simulink model "c230403_FCEV_SLMP_SQP"  (R2022b)
settings: Solver=FixedStepAuto  StartTime=0.0  StopTime=DrvCycLen  FixedStep=1  RelTol=1e-3
values from neighbouring files (symbols this model uses):
  AccThrshd = 1    [Config_c221112.m]    (also in Config_c221127.m; Config_c221218.m; Config_c230117.m; Config_c230321.m)
  AlphaRampFactor = 8    [Config_c221112.m]    (also in Config_c221127.m; Config_c221218.m; Config_c230117.m; Config_c230321.m)
  Bat_ori_SOC2 = [0 0.001 0.002 0.003 0.004 0.005 0.006 0.007 0.008 0.009 0.01 0.011 ... (1001 elements, 1x1001)]    [FCEV_original_data.mat]
  Bat_ori_Uoc_chg_V = [2.4478 2.54923264342 2.6007 2.6383 2.66953057366 2.69636321708 2.7197 2.74042850391 2.75906114733 2.77619379074 2.792 2.80675907757 ... (1001 elements, 1x1001)]    [FCEV_original_data.mat]
  Bat_ori_Uoc_dis_V = [1.9998 2.03916768329 2.24724374236 2.39700902919 2.48767431602 2.5476 2.5882 2.6202 2.64771773167 2.6719 2.6933 2.71251566192 ... (1001 elements, 1x1001)]    [FCEV_original_data.mat]
  Bat_power_max_kW = 50    [FCEV_original_data.mat]
  Bat_power_min_kW = 0    [FCEV_original_data.mat]
  Bat_SOC_min = 0.3    [FCEV_original_data.mat]
  BattOnly = 0    [Config_c221218.m]    (also in Config_c230117.m = BattSocRightNow > BattSocLowerLimit; Config_c230321.m = double(BattSocRightNow > BattSocLowerLimit))
  BattPack_current = BattCell_current * 9    (= 20.7)    [Config_c230321.m]
  BattSocInit = 0.9    [Config_c221112.m]    (also in Config_c221127.m = 0.3; Config_c221218.m = 0.3; Config_c230117.m = 0.8; Config_c230321.m = 0.8)
  BattSocLowerLimit = 0.25    [Config_c221112.m]    (also in Config_c221127.m = 0.3; Config_c221218.m = 0.3; Config_c230117.m = 0.3; Config_c230321.m = 0.3)
  BattSocRightNow = BattSocRightNow - SocDrop    [Config_c221218.m]    (also in Config_c230117.m; Config_c230321.m)
  BattSocUpperLimit = 0.9    [Config_c221112.m]    (also in Config_c221127.m = 0.8; Config_c221218.m = 0.8; Config_c230117.m = 0.8; Config_c230321.m = 0.8)
  CFWF = 0.5    [Config_c221127.m]    (also in Config_c221218.m; Config_c230117.m; Config_c230321.m)
  DCAC_eff = 0.95    [FCEV_original_data.mat]
  DCDC_ori_eff = [0.95 0.96 0.97 0.976 0.98 0.978 0.973 0.962]    [FCEV_original_data.mat]
  DCDC_ori_power_kW = [0 10 20 30 40 50 60 70]    [FCEV_original_data.mat]
  DeAccThrshd = -1    [Config_c221112.m]    (also in Config_c221127.m; Config_c221218.m; Config_c230117.m; Config_c230321.m)
  DeltaFcPwrRcm_down = 0.5    [Config_c221127.m]    (also in Config_c221218.m; Config_c230117.m; Config_c230321.m)
  DeltaFcPwrRcm_up = 2    [Config_c221127.m]    (also in Config_c221218.m = 3; Config_c230117.m = 4; Config_c230321.m = 4)
  DrvCycRange = sum(DrvCycVps(:,2))    [Config_c221112.m]    (also in Config_c221127.m; Config_c221218.m; Config_c230117.m; Config_c230321.m)
  FC_ori_eff = [0.1 0.33 0.492 0.533 0.559 0.596 0.591 0.562 0.508]    [FCEV_original_data.mat]
  FC_ori_fuel_rate_gps = [0 0.0505050505051 0.0846883468835 0.117260787992 0.149075730471 0.279642058166 0.423011844332 0.593119810202 0.820209973753]    [FCEV_original_data.mat]
  FC_ori_power_kW = [0 2 5 7.5 10 20 30 40 50]    [FCEV_original_data.mat]
  FC_power_max_kW = 50    [FCEV_original_data.mat]
  FC_power_min_kW = 0    [FCEV_original_data.mat]
  FcPwrDropCall = 6    [Config_c221127.m]    (also in Config_c221218.m; Config_c230117.m; Config_c230321.m)
  HydpriceRmb = 30    [Config_c221127.m]    (also in Config_c221218.m; Config_c230117.m; Config_c230321.m)
  m = Time_sample    [Config_c22100601.m]    (also in Config_c22100701.m)
  MC_eff_brk_average = 0.810578512397    [FCEV_original_data.mat]
  MC_eff_dri_average = 0.810578512397    [FCEV_original_data.mat]
  MC_inertia = 0.06    [FCEV_original_data.mat]
  MC_ori_eff = [0.7 0.78 0.85 0.86 0.81 0.82 0.79 0.78 0.78 0.78 0.78 0.7 ... (231 elements, 11x21)]    [FCEV_original_data.mat]
  MC_ori_power_brk_req_kW = [0 -28.3912930389 -56.7825860779 -85.1738791168 -113.565172156 -141.956465195 -170.347758234 -198.739051273 -227.130344311 -255.52163735 -283.912930389 0 ... (121 elements, 11x11)]    [FCEV_original_data.mat]
  MC_ori_power_dri_req_kW = [0 0 0 0 0 0 0 0 0 0 0 0 ... (121 elements, 11x11)]    [FCEV_original_data.mat]
  MC_ori_spd_rpm = [0 1000 2000 3000 4000 5000 6000 7000 8000 9000 10000]    [FCEV_original_data.mat]
  MC_ori_trq_brk_max_Nm = [-271.1368 -271.1368 -271.1368 -237.5159 -178.1369 -142.4824 -118.7579 -101.8119 -89.0685 -79.172 -71.1734]    [FCEV_original_data.mat]
  MC_ori_trq_brk_Nm = [-271.136848522 -244.02316367 -216.909478817 -189.795793965 -162.682109113 -135.568424261 -108.454739409 -81.3410545565 -54.2273697044 -27.1136848522 0]    [FCEV_original_data.mat]
  MC_ori_trq_dri_max_Nm = [271.1368 271.1368 271.1368 237.5159 178.1369 142.4824 118.7579 101.8119 89.0685 79.172 71.1734]    [FCEV_original_data.mat]
  MC_ori_trq_dri_Nm = [0 27.1136848522 54.2273697044 81.3410545565 108.454739409 135.568424261 162.682109113 189.795793965 216.909478817 244.02316367 271.136848522]    [FCEV_original_data.mat]
  MC_ori_trq_Nm = [-271.136848522 -244.02316367 -216.909478817 -189.795793965 -162.682109113 -135.568424261 -108.454739409 -81.3410545565 -54.2273697044 -27.1136848522 0 27.1136848522 ... (21 elements, 1x21)]    [FCEV_original_data.mat]
  MC_power_max_kW = 75    [FCEV_original_data.mat]
  MC_spd_max_rpm = 10000    [FCEV_original_data.mat]
  MC_spd_min_rpm = 0    [FCEV_original_data.mat]
  MC_spd_scale = 1    [FCEV_original_data.mat]
  MC_trq_scale = 1    [FCEV_original_data.mat]
  nbl_std = (20/nbl_btm)^(1/0.57)    [Config_c230321.m]
  no_FcPwrSlowDrop = 1    [Config_c230321.m]
  Placeholder = 0    [Config_c221127.m]    (also in Config_c221218.m; Config_c230117.m; Config_c230321.m)
  PredLen = 5    [Config_c221112.m]    (also in Config_c221127.m; Config_c221218.m; Config_c230117.m; Config_c230321.m)
  Q_batt = 20.7*3600    (= 74520)    [Config_c22100701.m]    (also in Config_c230321.m = 18000)
  Road_u = 0.75    [FCEV_original_data.mat]
  SC_np = 1    [Config_c230321.m]
  SC_ns = 100    [Config_c230321.m]
  SC_rc = 1000    [Config_c230321.m]
  SLMP_LearningRate = 0.05    [Config_c221112.m]    (also in Config_c221127.m; Config_c221218.m; Config_c230117.m; Config_c230321.m)
  tDegTable = [zeros(1,3),linspace(0,0.13,47)]    [Config_c221127.m]    (also in Config_c221218.m; Config_c230117.m; Config_c230321.m)
  usd2rmb = 7.116    [Config_c22100601.m]    (also in Config_c22100701.m; Config_c221106.m = 6; Config_c221112.m = 6; Config_c221127.m = 6)
  Veh_air_density_kgpm2 = 1.2    [FCEV_original_data.mat]
  Veh_brk_front = [1 0.6 0.608 0.61 0.618 0.624 0.636 0.645 0.655]    [FCEV_original_data.mat]
  Veh_brk_z = [0.1 0.2 0.3 0.4 0.5 0.6 0.7 0.8 0.9]    [FCEV_original_data.mat]
  Veh_brk_z_max = 0.7    [FCEV_original_data.mat]
  Veh_brk_z_min = 0.1    [FCEV_original_data.mat]
  Veh_coeff_drag = 0.312    [FCEV_original_data.mat]
  Veh_coeff_roll = 0.00863    [FCEV_original_data.mat]
  Veh_final_drive_inertia = 0.1105    [FCEV_original_data.mat]
  Veh_final_drive_ratio = 3.47    [FCEV_original_data.mat]
  Veh_frontal_area_m2 = 2.06    [FCEV_original_data.mat]
  Veh_gravity_acc_ms2 = 9.81    [FCEV_original_data.mat]
  Veh_mass_cargo_kg = 113    [FCEV_original_data.mat]
  Veh_mass_curb_kg = 1157    [FCEV_original_data.mat]
  Veh_mech_eff = 0.9    [FCEV_original_data.mat]
  Veh_rotary_mass_conversion_factor = 1.05    [FCEV_original_data.mat]
  Veh_size_cg_height_m = 0.53    [FCEV_original_data.mat]
  Veh_wheel_inertia = 3.1039    [FCEV_original_data.mat]
  Veh_wheel_radius_m = 0.313    [FCEV_original_data.mat]
  Veh_wt_frac_front = 0.5    [FCEV_original_data.mat]
  VstdThrshd = 2    [Config_c221112.m]    (also in Config_c221127.m; Config_c221218.m; Config_c230117.m; Config_c230321.m)
undefined symbols (not defined in the file or in its folder): Bat_ori_temp, SC_iv, SC_nm, SC_SocTable
libraries: autolibshared x2
(part 7 of 7)

== system c230403_FCEV_SLMP_SQP/Subsystem4/VehModel_Pred+9/车轮模型/Interia torque1 ==
  note: This block computes the torque required to overcome the inertia of the
      | wheels and axle.
  车轮线速度 m/s : Inport
  Add : Sum  Inputs=+-
  Add1 : Sum  Inputs=+-
  Clock : Clock
  Constant : Constant  Value=Veh_wheel_inertia
  Constant2 : Constant  Value=0
  Divide : Product  Inputs=**/
  Memory : Memory  InheritSampleTime=on
  Memory1 : Memory  InheritSampleTime=on
  Saturation : Saturate  UpperLimit=1.1  LowerLimit=0.9
  Switch : Switch  SaturateOnIntegerOverflow=off  InputSameDT=off
  axle input speed (rad/s) : Gain  Gain=1/Veh_wheel_radius_m
  inertia torque (Nm) : Outport  InitialOutput=0
  wires:
  Divide/1 -> inertia torque (Nm)/1
  车轮线速度 m/s/1 -> axle input speed (rad/s)/1
  Saturation/1 -> Divide/3
  Add1/1 -> Saturation/1
  Constant2/1 -> Switch/1
  axle input speed (rad/s)/1 -> Add/1, Memory/1
  Memory/1 -> Add/2
  Clock/1 -> Add1/1, Memory1/1
  Memory1/1 -> Add1/2
  Constant/1 -> Divide/2
  Add/1 -> Switch/3, Switch/2
  Switch/1 -> Divide/1

== system c230403_FCEV_SLMP_SQP/Subsystem4/VehModel_Pred+9/驱动电机模型/Brake torque_limited ==
  tor_req nm : Inport
  mc spd rpm : Inport  Port=2
  1-D Lookup Table : Lookup_n-D  NumberOfTableDimensions=1  BreakpointsForDimension1=MC_ori_spd_rpm  Table=MC_ori_trq_brk_max_Nm  RndMeth=Simplest
  MinMax : MinMax  Function=max  Inputs=2
  limted mc torque nm : Outport
  wires:
  MinMax/1 -> limted mc torque nm/1
  1-D Lookup Table/1 -> MinMax/2
  mc spd rpm/1 -> 1-D Lookup Table/1
  tor_req nm/1 -> MinMax/1

== system c230403_FCEV_SLMP_SQP/Subsystem4/VehModel_Pred+9/驱动电机模型/Drive torque_limited ==
  tor_req nm : Inport
  mc spd rpm : Inport  Port=2
  1-D Lookup Table : Lookup_n-D  NumberOfTableDimensions=1  BreakpointsForDimension1=MC_ori_spd_rpm  Table=MC_ori_trq_dri_max_Nm  RndMeth=Simplest
  MinMax : MinMax  Inputs=2
  limted mc torque nm : Outport
  wires:
  MinMax/1 -> limted mc torque nm/1
  1-D Lookup Table/1 -> MinMax/2
  mc spd rpm/1 -> 1-D Lookup Table/1
  tor_req nm/1 -> MinMax/1

== system c230403_FCEV_SLMP_SQP/Subsystem4/VehModel_Pred+9/驱动电机模型/Inertia torque ==
  motor spd rpm : Inport
  Derivative : Derivative
  Gain1 : Gain  Gain=MC_inertia
  rpm->rad/s : Gain  Gain=2*pi/60
  Out1 : Outport
  wires:
  motor spd rpm/1 -> rpm->rad/s/1
  rpm->rad/s/1 -> Derivative/1
  Gain1/1 -> Out1/1
  Derivative/1 -> Gain1/1

== system c230403_FCEV_SLMP_SQP/Subsystem4/VehModel_Pred+9/驱动电机模型/Inertia torque1 ==
  motor spd rpm : Inport
  Derivative : Derivative
  Gain1 : Gain  Gain=MC_inertia
  rpm->rad/s : Gain  Gain=2*pi/60
  Out1 : Outport
  wires:
  motor spd rpm/1 -> rpm->rad/s/1
  rpm->rad/s/1 -> Derivative/1
  Gain1/1 -> Out1/1
  Derivative/1 -> Gain1/1

== system c230403_FCEV_SLMP_SQP/VehModel_Current/车轮模型/Regenerative energy compute/compute of the brk energy ==
  motor brk force in front wheel N : Inport
  wheel linear spd m/s : Inport  Port=2
  Add : Sum
  Gain1 : Gain  Gain=-1
  Memory1 : Memory  InheritSampleTime=on
  Product : Product  RndMeth=Zero
  Scope : Scope
  Ws->kWh : Gain  Gain=1/(1000*3600)
  制动能量 : ToWorkspace  VariableName=Energy_regenerative_brk_kWh  SaveFormat=Timeseries  SampleTime=-1
  "regenerative brk energy kwh " : Outport
  wires:
  motor brk force in front wheel N/1 -> Product/1
  wheel linear spd m/s/1 -> Product/2
  Product/1 -> Gain1/1
  Ws->kWh/1 -> Scope/1, 制动能量/1, "regenerative brk energy kwh "/1
  Add/1 -> Memory1/1, Ws->kWh/1
  Memory1/1 -> Add/2
  Gain1/1 -> Add/1

== matlab function c230403_FCEV_SLMP_SQP/SuperCapacitor/MATLAB Function1 ==
  data: P input; y output; n input; c input; u_k input
function y = fcn(P,n,c,u_k)

y = (2*P/(n*c)+(u_k)^2)^(1/2);

== matlab function c230403_FCEV_SLMP_SQP/MATLAB Function ==
  data: PredLen input; Enable output
function Enable = fcn(PredLen)

u = zeros(9,1);
u(1:PredLen,1) = 1;

Enable = u;

== stateflow chart c230403_FCEV_SLMP_SQP/Chart ==
  state LowSpeed_URBAN
    note: [2,10]
    state LowConditioning
      entry:
      DrvState = 10;
    state LowDeAcc
      entry:
      DrvState = 9;
    state LowAcc
      entry:
      DrvState = 11;
    (default) -> LowConditioning
    LowConditioning -> (junction 81) [order 1] : [a_ave < DeAccThrshd]
    (junction 81) -> LowDeAcc : [v_std > VstdThrshd]
    LowDeAcc -> LowConditioning [order 1] : [a_ave > DeAccThrshd]
    LowDeAcc -> LowConditioning [order 2] : [v_std < VstdThrshd]
    LowConditioning -> (junction 78) [order 2] : [a_ave > AccThrshd]
    (junction 78) -> LowAcc : [v_std > VstdThrshd]
    LowAcc -> LowConditioning [order 2] : [a_ave < AccThrshd]
    LowAcc -> LowConditioning [order 1] : [v_std < VstdThrshd]
  state Init
    entry:
    DrvState = 0;
  state MidSpeed_SUBURB
    note: (10,25]
    state MidDeAcc
      entry:
      DrvState = 19;
    state MidConditioning
      entry:
      DrvState = 20;
    state MidAcc
      entry:
      DrvState = 21;
    (default) -> MidConditioning
    MidConditioning -> (junction 94) [order 1] : [a_ave < DeAccThrshd]
    (junction 94) -> MidDeAcc : [v_std > VstdThrshd]
    MidDeAcc -> MidConditioning [order 2] : [a_ave > DeAccThrshd]
    MidDeAcc -> MidConditioning [order 1] : [v_std < VstdThrshd]
    MidConditioning -> (junction 92) [order 2] : [a_ave > AccThrshd]
    (junction 92) -> MidAcc : [v_std > VstdThrshd]
    MidAcc -> MidConditioning [order 1] : [a_ave < AccThrshd]
    MidAcc -> MidConditioning [order 2] : [v_std < VstdThrshd]
  state HighSpeed_HIGHWAY
    note: (25,inf)
    state HighDeAcc
      entry:
      DrvState = 29;
    state HighConditioning
      entry:
      DrvState = 30;
    state HighAcc
      entry:
      DrvState = 31;
    (default) -> HighConditioning
    HighConditioning -> (junction 103) [order 1] : [a_ave < DeAccThrshd]
    (junction 103) -> HighDeAcc : [v_std > VstdThrshd]
    HighDeAcc -> HighConditioning [order 1] : [a_ave > DeAccThrshd]
    HighDeAcc -> HighConditioning [order 2] : [v_std < VstdThrshd]
    HighConditioning -> (junction 101) [order 2] : [a_ave > AccThrshd]
    (junction 101) -> HighAcc : [v_std > VstdThrshd]
    HighAcc -> HighConditioning [order 1] : [a_ave < AccThrshd]
    HighAcc -> HighConditioning [order 2] : [v_std < VstdThrshd]
  (default) -> Init
  Init -> LowSpeed_URBAN : [Vth_c2l <= v_ave && Vth_l2m >= v_ave]
  LowSpeed_URBAN -> Init [order 2] : [v_ave < Vth_c2l]
  MidSpeed_SUBURB -> LowSpeed_URBAN [order 1] : [Vth_c2l <= v_ave && Vth_l2m >= v_ave]
  LowSpeed_URBAN -> MidSpeed_SUBURB [order 1] : [Vth_l2m < v_ave && Vth_m2h >= v_ave]
  HighSpeed_HIGHWAY -> MidSpeed_SUBURB : [Vth_l2m < v_ave && Vth_m2h >= v_ave]
  MidSpeed_SUBURB -> HighSpeed_HIGHWAY [order 2] : [v_ave > Vth_m2h]
  data: DeAccThrshd parameter double; AccThrshd parameter double size=1; VstdThrshd parameter double size=5; v_std input; v_ave input; a_ave input; DrvState output; DeAccThrshd constant double [-10..0] =DeAccThrshd; AccThrshd constant double size=1 [0..10] =AccThrshd; VstdThrshd constant double size=4 =VstdThrshd; Vth_c2l constant double =Vth_c2l; Vth_l2m constant double =Vth_l2m; Vth_m2h constant double =Vth_m2h

== matlab function c230403_FCEV_SLMP_SQP/Subsystem3/FcDegCountingSubSys/MATLAB Function4 ==
  data: u input; y output; usd2rmb input
function y = FcDegHl(u,usd2rmb)
alpha_h = 10;   %10e-6V/h
u_eol = 100000;   %10e-6V
p_stack = 50*93*usd2rmb;

y = (alpha_h*p_stack/u_eol)*u/3600;

== matlab function c230403_FCEV_SLMP_SQP/Subsystem3/FcDegCountingSubSys/MATLAB Function5 ==
  data: u input; y output; usd2rmb input
function y = FcDegLl(u,usd2rmb)
alpha_l = 8.66;   %10e-6V/h
u_eol = 100000;   %10e-6V
p_stack = 50*93*usd2rmb;

y = (alpha_l*p_stack/u_eol)*u/3600;

== matlab function c230403_FCEV_SLMP_SQP/Subsystem3/FcDegCountingSubSys/MATLAB Function1 ==
  data: u input; y output
function y = FcDegLl_Logic(u)

if u > 0 && u <=10
    opt = 1;
else
    opt = 0;
end

y = opt;

== stateflow chart c230403_FCEV_SLMP_SQP/Subsystem10/Chart1 ==
  state Init
    entry:
    callopt = 0;
  state callup
    entry:
    callopt = 1;
  state calldown
    entry:
    callopt = 0;
  (default) -> Init
  callup -> calldown : [dropCall == 1]
  Init -> callup : [upCall == 1]
  calldown -> callup : [upCall == 1]
  data: upCall input boolean; dropCall input boolean; callopt output boolean
